simulink model "OcularMotorLabModel_2023_12_15_M22b"  (R2022b)
settings: Solver=FixedStepAuto  StartTime=tStart  StopTime=tFinal  FixedStep=0.001  RelTol=1e-3
undefined symbols (not defined in the file or in its folder): Asp, Asp1, Asp2, e0sp, gaussian, Gpc, GPos, Gsl, HeadToEye, IPD, psi, Psp1, RotFbk, SacThDeg, SatSp, sigbuilder_block, SomFbk, T1, T2, Tccanal, Tcn, Tcr, Tcsp, TCvs, tdm, tdsp1, tdsp2, tdsp3, tdv, Tsl, Tz, w
libraries: matrix_library x13, vrlib x9, simulink_extras x6, simulink x1
(part 2 of 2)

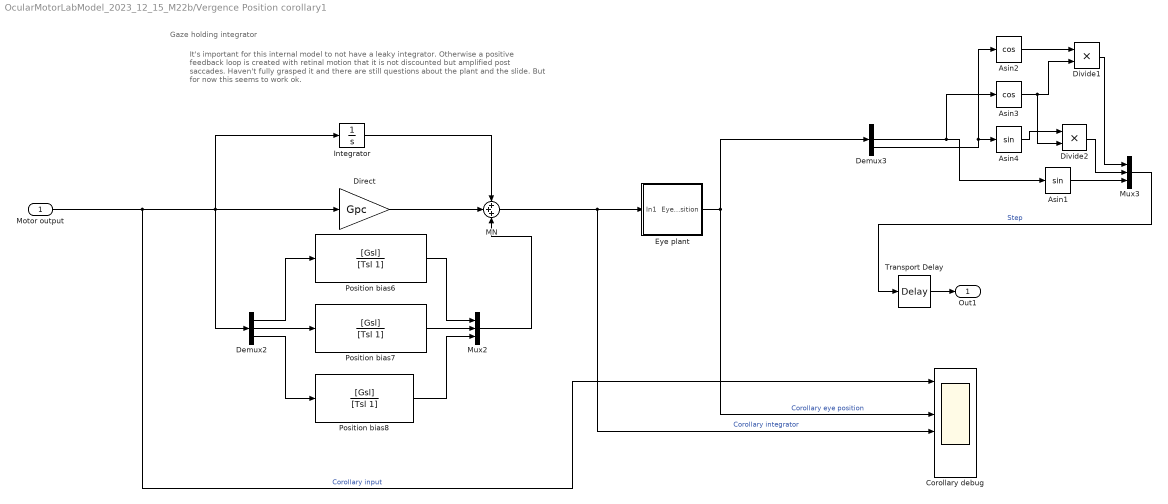
== system OcularMotorLabModel_2023_12_15_M22b/Vergence Position corollary1 ==
  note: Gaze holding integrator
  note: It's important for this internal model to not have a leaky integrator. Otherwise a positive feedback loop is created with retinal motion that it is not discounted but amplified post saccades.
      |
      | Haven't fully grasped it and there are still questions about the plant and the slide. But for now this seems to work ok.
  Motor output : Inport
  Asin1 : Trigonometry
  Asin2 : Trigonometry  Operator=cos
  Asin3 : Trigonometry  Operator=cos
  Asin4 : Trigonometry
  Corollary debug : Scope  NumInputPorts=6
  Demux2 : Demux  Outputs=3
  Demux3 : Demux  Outputs=3
  Direct : Gain  Gain=Gpc
  Divide1 : Product  Inputs=**
  Divide2 : Product  Inputs=**
  Eye plant : Subsystem
  Integrator : Integrator
  "MN " : Sum  Inputs=+++  InputSameDT=on  SaturateOnIntegerOverflow=on  OutDataTypeStr=Inherit: Same as first input
  Mux2 : Mux  Inputs=3
  Mux3 : Mux  Inputs=3
  Position bias6 : TransferFcn  Numerator=[Gsl]  Denominator=[Tsl 1]
  Position bias7 : TransferFcn  Numerator=[Gsl]  Denominator=[Tsl 1]
  Position bias8 : TransferFcn  Numerator=[Gsl]  Denominator=[Tsl 1]
  Transport Delay : TransportDelay  DelayTime=tdm
  Out1 : Outport
  wires:
  Motor output/1 -> Integrator/1, Direct/1, Demux2/1, Corollary debug/1  "Corollary input"
  Eye plant/1(Eye position) -> Demux3/1, Corollary debug/3  "Corollary eye position"
  "MN "/1 -> Eye plant/1(In1), Corollary debug/4  "Corollary integrator"
  Transport Delay/1 -> Out1/1
  Mux2/1 -> "MN "/3
  Integrator/1 -> "MN "/1
  Demux2/2 -> Position bias7/1
  Position bias8/1 -> Mux2/3
  Demux2/3 -> Position bias8/1
  Position bias6/1 -> Mux2/1
  Demux2/1 -> Position bias6/1
  Position bias7/1 -> Mux2/2
  Direct/1 -> "MN "/2
  Divide1/1 -> Mux3/1
  Asin1/1 -> Mux3/3
  Demux3/2 -> Asin3/1, Asin1/1
  Divide2/1 -> Mux3/2
  Asin3/1 -> Divide2/2, Divide1/2
  Asin2/1 -> Divide1/1
  Asin4/1 -> Divide2/1
  Demux3/3 -> Asin2/1, Asin4/1
  Mux3/1 -> Transport Delay/1  "Step"

== system OcularMotorLabModel_2023_12_15_M22b/Version ==
  Left : Inport
  Right : Inport  Port=2
  Constant : Constant  Value=2
  Divide : Product  Inputs=*/
  Sum : Sum  Inputs=|++
  Out1 : Outport
  wires:
  Divide/1 -> Out1/1
  Sum/1 -> Divide/1
  Left/1 -> Sum/1
  Constant/1 -> Divide/2
  Right/1 -> Sum/2

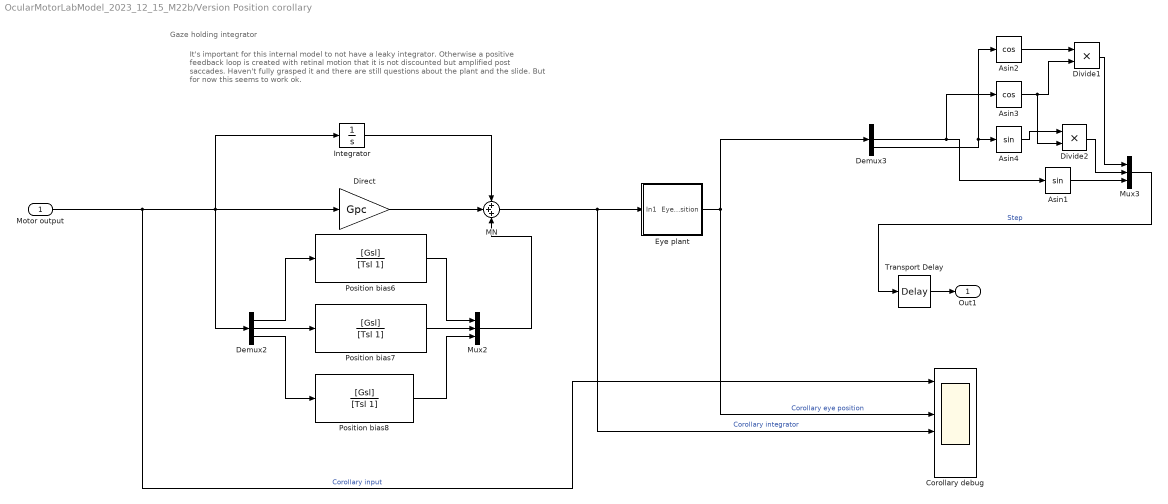
== system OcularMotorLabModel_2023_12_15_M22b/Version Position corollary ==
  note: Gaze holding integrator
  note: It's important for this internal model to not have a leaky integrator. Otherwise a positive feedback loop is created with retinal motion that it is not discounted but amplified post saccades.
      |
      | Haven't fully grasped it and there are still questions about the plant and the slide. But for now this seems to work ok.
  Motor output : Inport
  Asin1 : Trigonometry
  Asin2 : Trigonometry  Operator=cos
  Asin3 : Trigonometry  Operator=cos
  Asin4 : Trigonometry
  Corollary debug : Scope  NumInputPorts=6
  Demux2 : Demux  Outputs=3
  Demux3 : Demux  Outputs=3
  Direct : Gain  Gain=Gpc
  Divide1 : Product  Inputs=**
  Divide2 : Product  Inputs=**
  Eye plant : Subsystem
  Integrator : Integrator
  "MN " : Sum  Inputs=+++  InputSameDT=on  SaturateOnIntegerOverflow=on  OutDataTypeStr=Inherit: Same as first input
  Mux2 : Mux  Inputs=3
  Mux3 : Mux  Inputs=3
  Position bias6 : TransferFcn  Numerator=[Gsl]  Denominator=[Tsl 1]
  Position bias7 : TransferFcn  Numerator=[Gsl]  Denominator=[Tsl 1]
  Position bias8 : TransferFcn  Numerator=[Gsl]  Denominator=[Tsl 1]
  Transport Delay : TransportDelay  DelayTime=tdm
  Out1 : Outport
  wires:
  Motor output/1 -> Integrator/1, Direct/1, Demux2/1, Corollary debug/1  "Corollary input"
  Eye plant/1(Eye position) -> Demux3/1, Corollary debug/3  "Corollary eye position"
  "MN "/1 -> Eye plant/1(In1), Corollary debug/4  "Corollary integrator"
  Transport Delay/1 -> Out1/1
  Mux2/1 -> "MN "/3
  Integrator/1 -> "MN "/1
  Demux2/2 -> Position bias7/1
  Position bias8/1 -> Mux2/3
  Demux2/3 -> Position bias8/1
  Position bias6/1 -> Mux2/1
  Demux2/1 -> Position bias6/1
  Position bias7/1 -> Mux2/2
  Direct/1 -> "MN "/2
  Divide1/1 -> Mux3/1
  Asin1/1 -> Mux3/3
  Demux3/2 -> Asin3/1, Asin1/1
  Divide2/1 -> Mux3/2
  Asin3/1 -> Divide2/2, Divide1/2
  Asin2/1 -> Divide1/1
  Asin4/1 -> Divide2/1
  Demux3/3 -> Asin2/1, Asin4/1
  Mux3/1 -> Transport Delay/1  "Step"

== system OcularMotorLabModel_2023_12_15_M22b/Visual World Extrinsic Orientation (only for unidirectional reotations) ==
  Bus Creator : BusCreator  Tag=Bus Creator  Inputs=3
  FromWs : FromWorkspace  Tag=STV FromWs  VariableName=tuvar
      SigBuilderData=|
      | common.afterFinalStr = 'Extrapolate'
      | common.sampleTime = 0
      | dataSet(1).timeRange = [0 60]
      | dataSet(1).name = 'Roll 0.2 Hz'
      | dataSet(2).timeRange = [0 60]
      | dataSet(2).name = 'Roll 0.1 Hz'
      | dataSet(3).timeRange = [0 60]
      | dataSet(3).name = 'Roll 0.05 Hz'
      | dataSet(4).timeRange = [0 60]
      | dataSet(4).name = 'Roll 0.2 Hz IA'
      | dataSet(5).timeRange = [0 60]
      | dataSet(5).name = 'Roll 0.1 Hz IA'
      | dataSet(6).timeRange = [0 60]
      | dataSet(6).name = 'Roll 0.05 Hz IA'
      | dataSet(7).timeRange = [0 60]
      | dataSet(7).name = 'Roll 0.2 Hz RC'
      | dataSet(8).timeRange = [0 60]
      | dataSet(8).name = 'Roll 0.1 Hz RC'
      | dataSet(9).timeRange = [0 60]
      | dataSet(9).name = 'Roll 0.05 Hz RC'
      | dataSet(10).timeRange = [0 60]
      | dataSet(10).name = 'Zeros'
      | dataSet(11).timeRange = [0 60]
      | dataSet(11).name = 'SimpleSims'
      | sbobj.Groups(1).Name = 'Roll 0.2 Hz'
      | sbobj.Groups(1).Signals(1).Name = 'N-O (roll)'
      | sbobj.Groups(1).Signals(1).XData = [0 0.00500500500501 0.01001001001 0.015015015015 0.02002002002 0.025025025025 0.03003003003 0.035035035035 0.04004004004 0.045045045045 0.0500500500501 0.0550550550551 ... (11989 elements, 1x11989)]
      | sbobj.Groups(1).Signals(1).YData = [0 0.125788666321 0.251572356775 0.377346095689 0.503104907788 0.628843818382 0.754557853574 0.880242040448 1.00589140727 1.13150098368 1.25706580089 1.3825808919 ... (11989 elements, 1x11989)]
      | sbobj.Groups(1).Signals(2).Name = 'I-A (pitch)'
      | sbobj.Groups(1).Signals(2).XData = [0 60]
      | sbobj.Groups(1).Signals(2).YData = [0 0]
      | sbobj.Groups(1).Signals(3).Name = 'R-C (yaw)'
      | sbobj.Groups(1).Signals(3).XData = [0 60]
      | sbobj.Groups(1).Signals(3).YData = [0 0]
      | sbobj.Groups(1).TimeRange = [0 60]
      | sbobj.Groups(2).Name = 'Roll 0.1 Hz'
      | sbobj.Groups(2).Signals(1).Name = 'N-O (roll)'
      | sbobj.Groups(2).Signals(1).XData = [0 0.01001001001 0.02002002002 0.03003003003 0.04004004004 0.0500500500501 0.0600600600601 0.0700700700701 0.0800800800801 0.0900900900901 0.1001001001 0.11011011011 ... (5995 elements, 1x5995)]
      | sbobj.Groups(2).Signals(1).YData = [0 0.125788666321 0.251572356775 0.377346095689 0.503104907788 0.628843818382 0.754557853574 0.880242040448 1.00589140727 1.13150098368 1.25706580089 1.3825808919 ... (5995 elements, 1x5995)]
      | sbobj.Groups(2).Signals(2).Name = 'I-A (pitch)'
      | sbobj.Groups(2).Signals(2).XData = [0 60]
      | sbobj.Groups(2).Signals(2).YData = [0 0]
      | sbobj.Groups(2).Signals(3).Name = 'R-C (yaw)'
      | sbobj.Groups(2).Signals(3).XData = [0 60]
      | sbobj.Groups(2).Signals(3).YData = [0 0]
      | sbobj.Groups(2).TimeRange = [0 60]
      | sbobj.Groups(3).Name = 'Roll 0.05 Hz'
      | sbobj.Groups(3).Signals(1).Name = 'N-O (roll)'
      | sbobj.Groups(3).Signals(1).XData = [0 0.02002002002 0.04004004004 0.0600600600601 0.0800800800801 0.1001001001 0.12012012012 0.14014014014 0.16016016016 0.18018018018 0.2002002002 0.22022022022 ... (2998 elements, 1x2998)]
      | sbobj.Groups(3).Signals(1).YData = [0 0.125788666321 0.251572356775 0.377346095689 0.503104907788 0.628843818382 0.754557853574 0.880242040448 1.00589140727 1.13150098368 1.25706580089 1.3825808919 ... (2998 elements, 1x2998)]
      | sbobj.Groups(3).Signals(2).Name = 'I-A (pitch)'
      | sbobj.Groups(3).Signals(2).XData = [0 60]
      | sbobj.Groups(3).Signals(2).YData = [0 0]
      | sbobj.Groups(3).Signals(3).Name = 'R-C (yaw)'
      | sbobj.Groups(3).Signals(3).XData = [0 60]
      | sbobj.Groups(3).Signals(3).YData = [0 0]
      | sbobj.Groups(3).TimeRange = [0 60]
      | sbobj.Groups(4).Name = 'Roll 0.2 Hz IA'
      | sbobj.Groups(4).Signals(1).Name = 'N-O (roll)'
      | sbobj.Groups(4).Signals(1).XData = [0 60]
      | sbobj.Groups(4).Signals(1).YData = [0 0]
      | sbobj.Groups(4).Signals(2).Name = 'I-A (pitch)'
      | sbobj.Groups(4).Signals(2).XData = [0 0.00500500500501 0.01001001001 0.015015015015 0.02002002002 0.025025025025 0.03003003003 0.035035035035 0.04004004004 0.045045045045 0.0500500500501 0.0550550550551 ... (11989 elements, 1x11989)]
      | sbobj.Groups(4).Signals(2).YData = [0 0.125788666321 0.251572356775 0.377346095689 0.503104907788 0.628843818382 0.754557853574 0.880242040448 1.00589140727 1.13150098368 1.25706580089 1.3825808919 ... (11989 elements, 1x11989)]
      | sbobj.Groups(4).Signals(3).Name = 'R-C (yaw)'
      | sbobj.Groups(4).Signals(3).XData = [0 60]
      | sbobj.Groups(4).Signals(3).YData = [0 0]
      | sbobj.Groups(4).TimeRange = [0 60]
      | sbobj.Groups(5).Name = 'Roll 0.1 Hz IA'
      | sbobj.Groups(5).Signals(1).Name = 'N-O (roll)'
      | sbobj.Groups(5).Signals(1).XData = [0 60]
      | sbobj.Groups(5).Signals(1).YData = [0 0]
      | sbobj.Groups(5).Signals(2).Name = 'I-A (pitch)'
      | sbobj.Groups(5).Signals(2).XData = [0 0.01001001001 0.02002002002 0.03003003003 0.04004004004 0.0500500500501 0.0600600600601 0.0700700700701 0.0800800800801 0.0900900900901 0.1001001001 0.11011011011 ... (5995 elements, 1x5995)]
      | sbobj.Groups(5).Signals(2).YData = [0 0.125788666321 0.251572356775 0.377346095689 0.503104907788 0.628843818382 0.754557853574 0.880242040448 1.00589140727 1.13150098368 1.25706580089 1.3825808919 ... (5995 elements, 1x5995)]
      | sbobj.Groups(5).Signals(3).Name = 'R-C (yaw)'
      | sbobj.Groups(5).Signals(3).XData = [0 60]
      | sbobj.Groups(5).Signals(3).YData = [0 0]
      | sbobj.Groups(5).TimeRange = [0 60]
      | sbobj.Groups(6).Name = 'Roll 0.05 Hz IA'
      | sbobj.Groups(6).Signals(1).Name = 'N-O (roll)'
      | sbobj.Groups(6).Signals(1).XData = [0 60]
      | sbobj.Groups(6).Signals(1).YData = [0 0]
      | sbobj.Groups(6).Signals(2).Name = 'I-A (pitch)'
      | sbobj.Groups(6).Signals(2).XData = [0 0.02002002002 0.04004004004 0.0600600600601 0.0800800800801 0.1001001001 0.12012012012 0.14014014014 0.16016016016 0.18018018018 0.2002002002 0.22022022022 ... (2998 elements, 1x2998)]
      | sbobj.Groups(6).Signals(2).YData = [0 0.125788666321 0.251572356775 0.377346095689 0.503104907788 0.628843818382 0.754557853574 0.880242040448 1.00589140727 1.13150098368 1.25706580089 1.3825808919 ... (2998 elements, 1x2998)]
      | sbobj.Groups(6).Signals(3).Name = 'R-C (yaw)'
      | sbobj.Groups(6).Signals(3).XData = [0 60]
      | sbobj.Groups(6).Signals(3).YData = [0 0]
      | sbobj.Groups(6).TimeRange = [0 60]
      | sbobj.Groups(7).Name = 'Roll 0.2 Hz RC'
      | sbobj.Groups(7).Signals(1).Name = 'N-O (roll)'
      | sbobj.Groups(7).Signals(1).XData = [0 60]
      | sbobj.Groups(7).Signals(1).YData = [0 0]
      | sbobj.Groups(7).Signals(2).Name = 'I-A (pitch)'
      | sbobj.Groups(7).Signals(2).XData = [0 60]
      | sbobj.Groups(7).Signals(2).YData = [0 0]
      | sbobj.Groups(7).Signals(3).Name = 'R-C (yaw)'
      | sbobj.Groups(7).Signals(3).XData = [0 0.00500500500501 0.01001001001 0.015015015015 0.02002002002 0.025025025025 0.03003003003 0.035035035035 0.04004004004 0.045045045045 0.0500500500501 0.0550550550551 ... (11989 elements, 1x11989)]
      | sbobj.Groups(7).Signals(3).YData = [0 0.125788666321 0.251572356775 0.377346095689 0.503104907788 0.628843818382 0.754557853574 0.880242040448 1.00589140727 1.13150098368 1.25706580089 1.3825808919 ... (11989 elements, 1x11989)]
      | sbobj.Groups(7).TimeRange = [0 60]
      | sbobj.Groups(8).Name = 'Roll 0.1 Hz RC'
      | sbobj.Groups(8).Signals(1).Name = 'N-O (roll)'
      | sbobj.Groups(8).Signals(1).XData = [0 60]
      | sbobj.Groups(8).Signals(1).YData = [0 0]
      | sbobj.Groups(8).Signals(2).Name = 'I-A (pitch)'
      | sbobj.Groups(8).Signals(2).XData = [0 60]
      | sbobj.Groups(8).Signals(2).YData = [0 0]
      | sbobj.Groups(8).Signals(3).Name = 'R-C (yaw)'
      | sbobj.Groups(8).Signals(3).XData = [0 0.01001001001 0.02002002002 0.03003003003 0.04004004004 0.0500500500501 0.0600600600601 0.0700700700701 0.0800800800801 0.0900900900901 0.1001001001 0.11011011011 ... (5995 elements, 1x5995)]
      | sbobj.Groups(8).Signals(3).YData = [0 0.125788666321 0.251572356775 0.377346095689 0.503104907788 0.628843818382 0.754557853574 0.880242040448 1.00589140727 1.13150098368 1.25706580089 1.3825808919 ... (5995 elements, 1x5995)]
      | sbobj.Groups(8).TimeRange = [0 60]
      | sbobj.Groups(9).Name = 'Roll 0.05 Hz RC'
      | sbobj.Groups(9).Signals(1).Name = 'N-O (roll)'
      | sbobj.Groups(9).Signals(1).XData = [0 60]
      | sbobj.Groups(9).Signals(1).YData = [0 0]
      | sbobj.Groups(9).Signals(2).Name = 'I-A (pitch)'
      | sbobj.Groups(9).Signals(2).XData = [0 60]
      | sbobj.Groups(9).Signals(2).YData = [0 0]
      | sbobj.Groups(9).Signals(3).Name = 'R-C (yaw)'
      | sbobj.Groups(9).Signals(3).XData = [0 0.02002002002 0.04004004004 0.0600600600601 0.0800800800801 0.1001001001 0.12012012012 0.14014014014 0.16016016016 0.18018018018 0.2002002002 0.22022022022 ... (2998 elements, 1x2998)]
      | sbobj.Groups(9).Signals(3).YData = [0 0.125788666321 0.251572356775 0.377346095689 0.503104907788 0.628843818382 0.754557853574 0.880242040448 1.00589140727 1.13150098368 1.25706580089 1.3825808919 ... (2998 elements, 1x2998)]
      | sbobj.Groups(9).TimeRange = [0 60]
      | sbobj.Groups(10).Name = 'Zeros'
      | sbobj.Groups(10).Signals(1).Name = 'N-O (roll)'
      | sbobj.Groups(10).Signals(1).XData = [0 60]
      | sbobj.Groups(10).Signals(1).YData = [0 0]
      | sbobj.Groups(10).Signals(2).Name = 'I-A (pitch)'
      | sbobj.Groups(10).Signals(2).XData = [0 60]
      | sbobj.Groups(10).Signals(2).YData = [0 0]
      | sbobj.Groups(10).Signals(3).Name = 'R-C (yaw)'
      | sbobj.Groups(10).Signals(3).XData = [0 60]
      | sbobj.Groups(10).Signals(3).YData = [0 0]
      | sbobj.Groups(10).TimeRange = [0 60]
      | sbobj.Groups(11).Name = 'SimpleSims'
      | sbobj.Groups(11).Signals(1).Name = 'N-O (roll)'
      | sbobj.Groups(11).Signals(1).XData = [0 0.01 0.02 0.03 0.04 0.05 0.06 0.07 0.08 0.09 0.1 0.11 ... (6001 elements, 1x6001)]
      | sbobj.Groups(11).Signals(1).YData = [0 0.0628317497176 0.125662879311 0.188492768663 0.251320797667 0.314146346236 0.376968794308 0.43978752185 0.502601908867 0.565411335405 0.628215181563 0.691012827489 ... (6001 elements, 1x6001)]
      | sbobj.Groups(11).Signals(2).Name = 'I-A (pitch)'
      | sbobj.Groups(11).Signals(2).XData = [0 5 35 60]
      | sbobj.Groups(11).Signals(2).YData = [0 0 0 0]
      | sbobj.Groups(11).Signals(3).Name = 'R-C (yaw)'
      | sbobj.Groups(11).Signals(3).XData = [0 5 35 60]
      | sbobj.Groups(11).Signals(3).YData = [0 0 0 0]
      | sbobj.Groups(11).TimeRange = [0 60]
  Subsystem : Subsystem
  Bus : Outport
  wires:
  FromWs/1 -> Subsystem/1(In1)
  Subsystem/1(N-O (roll)) -> Bus Creator/1  "N-O (roll)"
  Subsystem/2(I-A (pitch)) -> Bus Creator/2  "I-A (pitch)"
  Subsystem/3(R-C (yaw)) -> Bus Creator/3  "R-C (yaw)"
  Bus Creator/1 -> Bus/1

== system OcularMotorLabModel_2023_12_15_M22b/Visual World Extrinsic velocity ==
  Bus Creator : BusCreator  Tag=Bus Creator  Inputs=3
  FromWs : FromWorkspace  Tag=STV FromWs  VariableName=tuvar
      SigBuilderData=|
      | common.afterFinalStr = 'Extrapolate'
      | common.sampleTime = 0
      | dataSet(1).timeRange = [0 60]
      | dataSet(1).name = 'Roll 0.2 Hz'
      | dataSet(2).timeRange = [0 60]
      | dataSet(2).name = 'Roll 0.1 Hz'
      | dataSet(3).timeRange = [0 60]
      | dataSet(3).name = 'Roll 0.05 Hz'
      | dataSet(4).timeRange = [0 60]
      | dataSet(4).name = 'Roll 0.2 Hz IA'
      | dataSet(5).timeRange = [0 60]
      | dataSet(5).name = 'Roll 0.1 Hz IA'
      | dataSet(6).timeRange = [0 60]
      | dataSet(6).name = 'Roll 0.05 Hz IA'
      | dataSet(7).timeRange = [0 60]
      | dataSet(7).name = 'Roll 0.2 Hz RC'
      | dataSet(8).timeRange = [0 60]
      | dataSet(8).name = 'Roll 0.1 Hz RC'
      | dataSet(9).timeRange = [0 60]
      | dataSet(9).name = 'Roll 0.05 Hz RC'
      | dataSet(10).timeRange = [0 60]
      | dataSet(10).name = 'Zeros'
      | dataSet(11).timeRange = [0 60]
      | dataSet(11).name = 'SimpleSims'
      | dataSet(12).timeRange = [0 60]
      | dataSet(12).name = 'YawOKN30degs'
      | sbobj.Groups(1).Name = 'Roll 0.2 Hz'
      | sbobj.Groups(1).Signals(1).Name = 'N-O (roll)'
      | sbobj.Groups(1).Signals(1).XData = [0 0.00500500500501 0.01001001001 0.015015015015 0.02002002002 0.025025025025 0.03003003003 0.035035035035 0.04004004004 0.045045045045 0.0500500500501 0.0550550550551 ... (11989 elements, 1x11989)]
      | sbobj.Groups(1).Signals(1).YData = [0 0.125788666321 0.251572356775 0.377346095689 0.503104907788 0.628843818382 0.754557853574 0.880242040448 1.00589140727 1.13150098368 1.25706580089 1.3825808919 ... (11989 elements, 1x11989)]
      | sbobj.Groups(1).Signals(2).Name = 'I-A (pitch)'
      | sbobj.Groups(1).Signals(2).XData = [0 60]
      | sbobj.Groups(1).Signals(2).YData = [0 0]
      | sbobj.Groups(1).Signals(3).Name = 'R-C (yaw)'
      | sbobj.Groups(1).Signals(3).XData = [0 60]
      | sbobj.Groups(1).Signals(3).YData = [0 0]
      | sbobj.Groups(1).TimeRange = [0 60]
      | sbobj.Groups(2).Name = 'Roll 0.1 Hz'
      | sbobj.Groups(2).Signals(1).Name = 'N-O (roll)'
      | sbobj.Groups(2).Signals(1).XData = [0 0.01001001001 0.02002002002 0.03003003003 0.04004004004 0.0500500500501 0.0600600600601 0.0700700700701 0.0800800800801 0.0900900900901 0.1001001001 0.11011011011 ... (5995 elements, 1x5995)]
      | sbobj.Groups(2).Signals(1).YData = [0 0.125788666321 0.251572356775 0.377346095689 0.503104907788 0.628843818382 0.754557853574 0.880242040448 1.00589140727 1.13150098368 1.25706580089 1.3825808919 ... (5995 elements, 1x5995)]
      | sbobj.Groups(2).Signals(2).Name = 'I-A (pitch)'
      | sbobj.Groups(2).Signals(2).XData = [0 60]
      | sbobj.Groups(2).Signals(2).YData = [0 0]
      | sbobj.Groups(2).Signals(3).Name = 'R-C (yaw)'
      | sbobj.Groups(2).Signals(3).XData = [0 60]
      | sbobj.Groups(2).Signals(3).YData = [0 0]
      | sbobj.Groups(2).TimeRange = [0 60]
      | sbobj.Groups(3).Name = 'Roll 0.05 Hz'
      | sbobj.Groups(3).Signals(1).Name = 'N-O (roll)'
      | sbobj.Groups(3).Signals(1).XData = [0 0.02002002002 0.04004004004 0.0600600600601 0.0800800800801 0.1001001001 0.12012012012 0.14014014014 0.16016016016 0.18018018018 0.2002002002 0.22022022022 ... (2998 elements, 1x2998)]
      | sbobj.Groups(3).Signals(1).YData = [0 0.125788666321 0.251572356775 0.377346095689 0.503104907788 0.628843818382 0.754557853574 0.880242040448 1.00589140727 1.13150098368 1.25706580089 1.3825808919 ... (2998 elements, 1x2998)]
      | sbobj.Groups(3).Signals(2).Name = 'I-A (pitch)'
      | sbobj.Groups(3).Signals(2).XData = [0 60]
      | sbobj.Groups(3).Signals(2).YData = [0 0]
      | sbobj.Groups(3).Signals(3).Name = 'R-C (yaw)'
      | sbobj.Groups(3).Signals(3).XData = [0 60]
      | sbobj.Groups(3).Signals(3).YData = [0 0]
      | sbobj.Groups(3).TimeRange = [0 60]
      | sbobj.Groups(4).Name = 'Roll 0.2 Hz IA'
      | sbobj.Groups(4).Signals(1).Name = 'N-O (roll)'
      | sbobj.Groups(4).Signals(1).XData = [0 60]
      | sbobj.Groups(4).Signals(1).YData = [0 0]
      | sbobj.Groups(4).Signals(2).Name = 'I-A (pitch)'
      | sbobj.Groups(4).Signals(2).XData = [0 0.00500500500501 0.01001001001 0.015015015015 0.02002002002 0.025025025025 0.03003003003 0.035035035035 0.04004004004 0.045045045045 0.0500500500501 0.0550550550551 ... (11989 elements, 1x11989)]
      | sbobj.Groups(4).Signals(2).YData = [0 0.125788666321 0.251572356775 0.377346095689 0.503104907788 0.628843818382 0.754557853574 0.880242040448 1.00589140727 1.13150098368 1.25706580089 1.3825808919 ... (11989 elements, 1x11989)]
      | sbobj.Groups(4).Signals(3).Name = 'R-C (yaw)'
      | sbobj.Groups(4).Signals(3).XData = [0 60]
      | sbobj.Groups(4).Signals(3).YData = [0 0]
      | sbobj.Groups(4).TimeRange = [0 60]
      | sbobj.Groups(5).Name = 'Roll 0.1 Hz IA'
      | sbobj.Groups(5).Signals(1).Name = 'N-O (roll)'
      | sbobj.Groups(5).Signals(1).XData = [0 60]
      | sbobj.Groups(5).Signals(1).YData = [0 0]
      | sbobj.Groups(5).Signals(2).Name = 'I-A (pitch)'
      | sbobj.Groups(5).Signals(2).XData = [0 0.01001001001 0.02002002002 0.03003003003 0.04004004004 0.0500500500501 0.0600600600601 0.0700700700701 0.0800800800801 0.0900900900901 0.1001001001 0.11011011011 ... (5995 elements, 1x5995)]
      | sbobj.Groups(5).Signals(2).YData = [0 0.125788666321 0.251572356775 0.377346095689 0.503104907788 0.628843818382 0.754557853574 0.880242040448 1.00589140727 1.13150098368 1.25706580089 1.3825808919 ... (5995 elements, 1x5995)]
      | sbobj.Groups(5).Signals(3).Name = 'R-C (yaw)'
      | sbobj.Groups(5).Signals(3).XData = [0 60]
      | sbobj.Groups(5).Signals(3).YData = [0 0]
      | sbobj.Groups(5).TimeRange = [0 60]
      | sbobj.Groups(6).Name = 'Roll 0.05 Hz IA'
      | sbobj.Groups(6).Signals(1).Name = 'N-O (roll)'
      | sbobj.Groups(6).Signals(1).XData = [0 60]
      | sbobj.Groups(6).Signals(1).YData = [0 0]
      | sbobj.Groups(6).Signals(2).Name = 'I-A (pitch)'
      | sbobj.Groups(6).Signals(2).XData = [0 0.02002002002 0.04004004004 0.0600600600601 0.0800800800801 0.1001001001 0.12012012012 0.14014014014 0.16016016016 0.18018018018 0.2002002002 0.22022022022 ... (2998 elements, 1x2998)]
      | sbobj.Groups(6).Signals(2).YData = [0 0.125788666321 0.251572356775 0.377346095689 0.503104907788 0.628843818382 0.754557853574 0.880242040448 1.00589140727 1.13150098368 1.25706580089 1.3825808919 ... (2998 elements, 1x2998)]
      | sbobj.Groups(6).Signals(3).Name = 'R-C (yaw)'
      | sbobj.Groups(6).Signals(3).XData = [0 60]
      | sbobj.Groups(6).Signals(3).YData = [0 0]
      | sbobj.Groups(6).TimeRange = [0 60]
      | sbobj.Groups(7).Name = 'Roll 0.2 Hz RC'
      | sbobj.Groups(7).Signals(1).Name = 'N-O (roll)'
      | sbobj.Groups(7).Signals(1).XData = [0 60]
      | sbobj.Groups(7).Signals(1).YData = [0 0]
      | sbobj.Groups(7).Signals(2).Name = 'I-A (pitch)'
      | sbobj.Groups(7).Signals(2).XData = [0 60]
      | sbobj.Groups(7).Signals(2).YData = [0 0]
      | sbobj.Groups(7).Signals(3).Name = 'R-C (yaw)'
      | sbobj.Groups(7).Signals(3).XData = [0 0.00500500500501 0.01001001001 0.015015015015 0.02002002002 0.025025025025 0.03003003003 0.035035035035 0.04004004004 0.045045045045 0.0500500500501 0.0550550550551 ... (11989 elements, 1x11989)]
      | sbobj.Groups(7).Signals(3).YData = [0 0.125788666321 0.251572356775 0.377346095689 0.503104907788 0.628843818382 0.754557853574 0.880242040448 1.00589140727 1.13150098368 1.25706580089 1.3825808919 ... (11989 elements, 1x11989)]
      | sbobj.Groups(7).TimeRange = [0 60]
      | sbobj.Groups(8).Name = 'Roll 0.1 Hz RC'
      | sbobj.Groups(8).Signals(1).Name = 'N-O (roll)'
      | sbobj.Groups(8).Signals(1).XData = [0 60]
      | sbobj.Groups(8).Signals(1).YData = [0 0]
      | sbobj.Groups(8).Signals(2).Name = 'I-A (pitch)'
      | sbobj.Groups(8).Signals(2).XData = [0 60]
      | sbobj.Groups(8).Signals(2).YData = [0 0]
      | sbobj.Groups(8).Signals(3).Name = 'R-C (yaw)'
      | sbobj.Groups(8).Signals(3).XData = [0 0.01001001001 0.02002002002 0.03003003003 0.04004004004 0.0500500500501 0.0600600600601 0.0700700700701 0.0800800800801 0.0900900900901 0.1001001001 0.11011011011 ... (5995 elements, 1x5995)]
      | sbobj.Groups(8).Signals(3).YData = [0 0.125788666321 0.251572356775 0.377346095689 0.503104907788 0.628843818382 0.754557853574 0.880242040448 1.00589140727 1.13150098368 1.25706580089 1.3825808919 ... (5995 elements, 1x5995)]
      | sbobj.Groups(8).TimeRange = [0 60]
      | sbobj.Groups(9).Name = 'Roll 0.05 Hz RC'
      | sbobj.Groups(9).Signals(1).Name = 'N-O (roll)'
      | sbobj.Groups(9).Signals(1).XData = [0 60]
      | sbobj.Groups(9).Signals(1).YData = [0 0]
      | sbobj.Groups(9).Signals(2).Name = 'I-A (pitch)'
      | sbobj.Groups(9).Signals(2).XData = [0 60]
      | sbobj.Groups(9).Signals(2).YData = [0 0]
      | sbobj.Groups(9).Signals(3).Name = 'R-C (yaw)'
      | sbobj.Groups(9).Signals(3).XData = [0 0.02002002002 0.04004004004 0.0600600600601 0.0800800800801 0.1001001001 0.12012012012 0.14014014014 0.16016016016 0.18018018018 0.2002002002 0.22022022022 ... (2998 elements, 1x2998)]
      | sbobj.Groups(9).Signals(3).YData = [0 0.125788666321 0.251572356775 0.377346095689 0.503104907788 0.628843818382 0.754557853574 0.880242040448 1.00589140727 1.13150098368 1.25706580089 1.3825808919 ... (2998 elements, 1x2998)]
      | sbobj.Groups(9).TimeRange = [0 60]
      | sbobj.Groups(10).Name = 'Zeros'
      | sbobj.Groups(10).Signals(1).Name = 'N-O (roll)'
      | sbobj.Groups(10).Signals(1).XData = [0 60]
      | sbobj.Groups(10).Signals(1).YData = [0 0]
      | sbobj.Groups(10).Signals(2).Name = 'I-A (pitch)'
      | sbobj.Groups(10).Signals(2).XData = [0 60]
      | sbobj.Groups(10).Signals(2).YData = [0 0]
      | sbobj.Groups(10).Signals(3).Name = 'R-C (yaw)'
      | sbobj.Groups(10).Signals(3).XData = [0 60]
      | sbobj.Groups(10).Signals(3).YData = [0 0]
      | sbobj.Groups(10).TimeRange = [0 60]
      | sbobj.Groups(11).Name = 'SimpleSims'
      | sbobj.Groups(11).Signals(1).Name = 'N-O (roll)'
      | sbobj.Groups(11).Signals(1).XData = [0 0.01 0.02 0.03 0.04 0.05 0.06 0.07 0.08 0.09 0.1 0.11 ... (6001 elements, 1x6001)]
      | sbobj.Groups(11).Signals(1).YData = [0 0.0628317497176 0.125662879311 0.188492768663 0.251320797667 0.314146346236 0.376968794308 0.43978752185 0.502601908867 0.565411335405 0.628215181563 0.691012827489 ... (6001 elements, 1x6001)]
      | sbobj.Groups(11).Signals(2).Name = 'I-A (pitch)'
      | sbobj.Groups(11).Signals(2).XData = [0 5 35 60]
      | sbobj.Groups(11).Signals(2).YData = [0 0 0 0]
      | sbobj.Groups(11).Signals(3).Name = 'R-C (yaw)'
      | sbobj.Groups(11).Signals(3).XData = [0 5 35 60]
      | sbobj.Groups(11).Signals(3).YData = [0 0 0 0]
      | sbobj.Groups(11).TimeRange = [0 60]
      | sbobj.Groups(12).Name = 'YawOKN30degs'
      | sbobj.Groups(12).Signals(1).Name = 'N-O (roll)'
      | sbobj.Groups(12).Signals(1).XData = [0 60]
      | sbobj.Groups(12).Signals(1).YData = [0 0]
      | sbobj.Groups(12).Signals(2).Name = 'I-A (pitch)'
      | sbobj.Groups(12).Signals(2).XData = [0 60]
      | sbobj.Groups(12).Signals(2).YData = [0 0]
      | sbobj.Groups(12).Signals(3).Name = 'R-C (yaw)'
      | sbobj.Groups(12).Signals(3).XData = [0 10 10 40.05 40.05 60]
      | sbobj.Groups(12).Signals(3).YData = [0 0 30 30 0 0]
      | sbobj.Groups(12).TimeRange = [0 60]
  Subsystem : Subsystem
  Bus : Outport
  wires:
  FromWs/1 -> Subsystem/1(In1)
  Subsystem/1(N-O (roll)) -> Bus Creator/1  "N-O (roll)"
  Subsystem/2(I-A (pitch)) -> Bus Creator/2  "I-A (pitch)"
  Subsystem/3(R-C (yaw)) -> Bus Creator/3  "R-C (yaw)"
  Bus Creator/1 -> Bus/1

== system OcularMotorLabModel_2023_12_15_M22b/Visual World Intrinsic velocity ==
  Bus Creator : BusCreator  Tag=Bus Creator  Inputs=3
  FromWs : FromWorkspace  Tag=STV FromWs  VariableName=tuvar
      SigBuilderData=|
      | common.afterFinalStr = 'Extrapolate'
      | common.sampleTime = 0
      | dataSet(1).timeRange = [0 60]
      | dataSet(1).name = 'Roll 0.2 Hz'
      | dataSet(2).timeRange = [0 60]
      | dataSet(2).name = 'Roll 0.1 Hz'
      | dataSet(3).timeRange = [0 60]
      | dataSet(3).name = 'Roll 0.05 Hz'
      | dataSet(4).timeRange = [0 60]
      | dataSet(4).name = 'Roll 0.2 Hz IA'
      | dataSet(5).timeRange = [0 60]
      | dataSet(5).name = 'Roll 0.1 Hz IA'
      | dataSet(6).timeRange = [0 60]
      | dataSet(6).name = 'Roll 0.05 Hz IA'
      | dataSet(7).timeRange = [0 60]
      | dataSet(7).name = 'Roll 0.2 Hz RC'
      | dataSet(8).timeRange = [0 60]
      | dataSet(8).name = 'Roll 0.1 Hz RC'
      | dataSet(9).timeRange = [0 60]
      | dataSet(9).name = 'Roll 0.05 Hz RC'
      | dataSet(10).timeRange = [0 60]
      | dataSet(10).name = 'Zeros'
      | dataSet(11).timeRange = [0 60]
      | dataSet(11).name = 'SimpleSims'
      | dataSet(12).timeRange = [0 60]
      | dataSet(12).name = 'YawOKN30degs'
      | sbobj.Groups(1).Name = 'Roll 0.2 Hz'
      | sbobj.Groups(1).Signals(1).Name = 'N-O (roll)'
      | sbobj.Groups(1).Signals(1).XData = [0 0.00500500500501 0.01001001001 0.015015015015 0.02002002002 0.025025025025 0.03003003003 0.035035035035 0.04004004004 0.045045045045 0.0500500500501 0.0550550550551 ... (11989 elements, 1x11989)]
      | sbobj.Groups(1).Signals(1).YData = [0 0.125788666321 0.251572356775 0.377346095689 0.503104907788 0.628843818382 0.754557853574 0.880242040448 1.00589140727 1.13150098368 1.25706580089 1.3825808919 ... (11989 elements, 1x11989)]
      | sbobj.Groups(1).Signals(2).Name = 'I-A (pitch)'
      | sbobj.Groups(1).Signals(2).XData = [0 60]
      | sbobj.Groups(1).Signals(2).YData = [0 0]
      | sbobj.Groups(1).Signals(3).Name = 'R-C (yaw)'
      | sbobj.Groups(1).Signals(3).XData = [0 60]
      | sbobj.Groups(1).Signals(3).YData = [0 0]
      | sbobj.Groups(1).TimeRange = [0 60]
      | sbobj.Groups(2).Name = 'Roll 0.1 Hz'
      | sbobj.Groups(2).Signals(1).Name = 'N-O (roll)'
      | sbobj.Groups(2).Signals(1).XData = [0 0.01001001001 0.02002002002 0.03003003003 0.04004004004 0.0500500500501 0.0600600600601 0.0700700700701 0.0800800800801 0.0900900900901 0.1001001001 0.11011011011 ... (5995 elements, 1x5995)]
      | sbobj.Groups(2).Signals(1).YData = [0 0.125788666321 0.251572356775 0.377346095689 0.503104907788 0.628843818382 0.754557853574 0.880242040448 1.00589140727 1.13150098368 1.25706580089 1.3825808919 ... (5995 elements, 1x5995)]
      | sbobj.Groups(2).Signals(2).Name = 'I-A (pitch)'
      | sbobj.Groups(2).Signals(2).XData = [0 60]
      | sbobj.Groups(2).Signals(2).YData = [0 0]
      | sbobj.Groups(2).Signals(3).Name = 'R-C (yaw)'
      | sbobj.Groups(2).Signals(3).XData = [0 60]
      | sbobj.Groups(2).Signals(3).YData = [0 0]
      | sbobj.Groups(2).TimeRange = [0 60]
      | sbobj.Groups(3).Name = 'Roll 0.05 Hz'
      | sbobj.Groups(3).Signals(1).Name = 'N-O (roll)'
      | sbobj.Groups(3).Signals(1).XData = [0 0.02002002002 0.04004004004 0.0600600600601 0.0800800800801 0.1001001001 0.12012012012 0.14014014014 0.16016016016 0.18018018018 0.2002002002 0.22022022022 ... (2998 elements, 1x2998)]
      | sbobj.Groups(3).Signals(1).YData = [0 0.125788666321 0.251572356775 0.377346095689 0.503104907788 0.628843818382 0.754557853574 0.880242040448 1.00589140727 1.13150098368 1.25706580089 1.3825808919 ... (2998 elements, 1x2998)]
      | sbobj.Groups(3).Signals(2).Name = 'I-A (pitch)'
      | sbobj.Groups(3).Signals(2).XData = [0 60]
      | sbobj.Groups(3).Signals(2).YData = [0 0]
      | sbobj.Groups(3).Signals(3).Name = 'R-C (yaw)'
      | sbobj.Groups(3).Signals(3).XData = [0 60]
      | sbobj.Groups(3).Signals(3).YData = [0 0]
      | sbobj.Groups(3).TimeRange = [0 60]
      | sbobj.Groups(4).Name = 'Roll 0.2 Hz IA'
      | sbobj.Groups(4).Signals(1).Name = 'N-O (roll)'
      | sbobj.Groups(4).Signals(1).XData = [0 60]
      | sbobj.Groups(4).Signals(1).YData = [0 0]
      | sbobj.Groups(4).Signals(2).Name = 'I-A (pitch)'
      | sbobj.Groups(4).Signals(2).XData = [0 0.00500500500501 0.01001001001 0.015015015015 0.02002002002 0.025025025025 0.03003003003 0.035035035035 0.04004004004 0.045045045045 0.0500500500501 0.0550550550551 ... (11989 elements, 1x11989)]
      | sbobj.Groups(4).Signals(2).YData = [0 0.125788666321 0.251572356775 0.377346095689 0.503104907788 0.628843818382 0.754557853574 0.880242040448 1.00589140727 1.13150098368 1.25706580089 1.3825808919 ... (11989 elements, 1x11989)]
      | sbobj.Groups(4).Signals(3).Name = 'R-C (yaw)'
      | sbobj.Groups(4).Signals(3).XData = [0 60]
      | sbobj.Groups(4).Signals(3).YData = [0 0]
      | sbobj.Groups(4).TimeRange = [0 60]
      | sbobj.Groups(5).Name = 'Roll 0.1 Hz IA'
      | sbobj.Groups(5).Signals(1).Name = 'N-O (roll)'
      | sbobj.Groups(5).Signals(1).XData = [0 60]
      | sbobj.Groups(5).Signals(1).YData = [0 0]
      | sbobj.Groups(5).Signals(2).Name = 'I-A (pitch)'
      | sbobj.Groups(5).Signals(2).XData = [0 0.01001001001 0.02002002002 0.03003003003 0.04004004004 0.0500500500501 0.0600600600601 0.0700700700701 0.0800800800801 0.0900900900901 0.1001001001 0.11011011011 ... (5995 elements, 1x5995)]
      | sbobj.Groups(5).Signals(2).YData = [0 0.125788666321 0.251572356775 0.377346095689 0.503104907788 0.628843818382 0.754557853574 0.880242040448 1.00589140727 1.13150098368 1.25706580089 1.3825808919 ... (5995 elements, 1x5995)]
      | sbobj.Groups(5).Signals(3).Name = 'R-C (yaw)'
      | sbobj.Groups(5).Signals(3).XData = [0 60]
      | sbobj.Groups(5).Signals(3).YData = [0 0]
      | sbobj.Groups(5).TimeRange = [0 60]
      | sbobj.Groups(6).Name = 'Roll 0.05 Hz IA'
      | sbobj.Groups(6).Signals(1).Name = 'N-O (roll)'
      | sbobj.Groups(6).Signals(1).XData = [0 60]
      | sbobj.Groups(6).Signals(1).YData = [0 0]
      | sbobj.Groups(6).Signals(2).Name = 'I-A (pitch)'
      | sbobj.Groups(6).Signals(2).XData = [0 0.02002002002 0.04004004004 0.0600600600601 0.0800800800801 0.1001001001 0.12012012012 0.14014014014 0.16016016016 0.18018018018 0.2002002002 0.22022022022 ... (2998 elements, 1x2998)]
      | sbobj.Groups(6).Signals(2).YData = [0 0.125788666321 0.251572356775 0.377346095689 0.503104907788 0.628843818382 0.754557853574 0.880242040448 1.00589140727 1.13150098368 1.25706580089 1.3825808919 ... (2998 elements, 1x2998)]
      | sbobj.Groups(6).Signals(3).Name = 'R-C (yaw)'
      | sbobj.Groups(6).Signals(3).XData = [0 60]
      | sbobj.Groups(6).Signals(3).YData = [0 0]
      | sbobj.Groups(6).TimeRange = [0 60]
      | sbobj.Groups(7).Name = 'Roll 0.2 Hz RC'
      | sbobj.Groups(7).Signals(1).Name = 'N-O (roll)'
      | sbobj.Groups(7).Signals(1).XData = [0 60]
      | sbobj.Groups(7).Signals(1).YData = [0 0]
      | sbobj.Groups(7).Signals(2).Name = 'I-A (pitch)'
      | sbobj.Groups(7).Signals(2).XData = [0 60]
      | sbobj.Groups(7).Signals(2).YData = [0 0]
      | sbobj.Groups(7).Signals(3).Name = 'R-C (yaw)'
      | sbobj.Groups(7).Signals(3).XData = [0 0.00500500500501 0.01001001001 0.015015015015 0.02002002002 0.025025025025 0.03003003003 0.035035035035 0.04004004004 0.045045045045 0.0500500500501 0.0550550550551 ... (11989 elements, 1x11989)]
      | sbobj.Groups(7).Signals(3).YData = [0 0.125788666321 0.251572356775 0.377346095689 0.503104907788 0.628843818382 0.754557853574 0.880242040448 1.00589140727 1.13150098368 1.25706580089 1.3825808919 ... (11989 elements, 1x11989)]
      | sbobj.Groups(7).TimeRange = [0 60]
      | sbobj.Groups(8).Name = 'Roll 0.1 Hz RC'
      | sbobj.Groups(8).Signals(1).Name = 'N-O (roll)'
      | sbobj.Groups(8).Signals(1).XData = [0 60]
      | sbobj.Groups(8).Signals(1).YData = [0 0]
      | sbobj.Groups(8).Signals(2).Name = 'I-A (pitch)'
      | sbobj.Groups(8).Signals(2).XData = [0 60]
      | sbobj.Groups(8).Signals(2).YData = [0 0]
      | sbobj.Groups(8).Signals(3).Name = 'R-C (yaw)'
      | sbobj.Groups(8).Signals(3).XData = [0 0.01001001001 0.02002002002 0.03003003003 0.04004004004 0.0500500500501 0.0600600600601 0.0700700700701 0.0800800800801 0.0900900900901 0.1001001001 0.11011011011 ... (5995 elements, 1x5995)]
      | sbobj.Groups(8).Signals(3).YData = [0 0.125788666321 0.251572356775 0.377346095689 0.503104907788 0.628843818382 0.754557853574 0.880242040448 1.00589140727 1.13150098368 1.25706580089 1.3825808919 ... (5995 elements, 1x5995)]
      | sbobj.Groups(8).TimeRange = [0 60]
      | sbobj.Groups(9).Name = 'Roll 0.05 Hz RC'
      | sbobj.Groups(9).Signals(1).Name = 'N-O (roll)'
      | sbobj.Groups(9).Signals(1).XData = [0 60]
      | sbobj.Groups(9).Signals(1).YData = [0 0]
      | sbobj.Groups(9).Signals(2).Name = 'I-A (pitch)'
      | sbobj.Groups(9).Signals(2).XData = [0 60]
      | sbobj.Groups(9).Signals(2).YData = [0 0]
      | sbobj.Groups(9).Signals(3).Name = 'R-C (yaw)'
      | sbobj.Groups(9).Signals(3).XData = [0 0.02002002002 0.04004004004 0.0600600600601 0.0800800800801 0.1001001001 0.12012012012 0.14014014014 0.16016016016 0.18018018018 0.2002002002 0.22022022022 ... (2998 elements, 1x2998)]
      | sbobj.Groups(9).Signals(3).YData = [0 0.125788666321 0.251572356775 0.377346095689 0.503104907788 0.628843818382 0.754557853574 0.880242040448 1.00589140727 1.13150098368 1.25706580089 1.3825808919 ... (2998 elements, 1x2998)]
      | sbobj.Groups(9).TimeRange = [0 60]
      | sbobj.Groups(10).Name = 'Zeros'
      | sbobj.Groups(10).Signals(1).Name = 'N-O (roll)'
      | sbobj.Groups(10).Signals(1).XData = [0 60]
      | sbobj.Groups(10).Signals(1).YData = [0 0]
      | sbobj.Groups(10).Signals(2).Name = 'I-A (pitch)'
      | sbobj.Groups(10).Signals(2).XData = [0 60]
      | sbobj.Groups(10).Signals(2).YData = [0 0]
      | sbobj.Groups(10).Signals(3).Name = 'R-C (yaw)'
      | sbobj.Groups(10).Signals(3).XData = [0 60]
      | sbobj.Groups(10).Signals(3).YData = [0 0]
      | sbobj.Groups(10).TimeRange = [0 60]
      | sbobj.Groups(11).Name = 'SimpleSims'
      | sbobj.Groups(11).Signals(1).Name = 'N-O (roll)'
      | sbobj.Groups(11).Signals(1).XData = [0 0.01 0.02 0.03 0.04 0.05 0.06 0.07 0.08 0.09 0.1 0.11 ... (6001 elements, 1x6001)]
      | sbobj.Groups(11).Signals(1).YData = [0 0.0628317497176 0.125662879311 0.188492768663 0.251320797667 0.314146346236 0.376968794308 0.43978752185 0.502601908867 0.565411335405 0.628215181563 0.691012827489 ... (6001 elements, 1x6001)]
      | sbobj.Groups(11).Signals(2).Name = 'I-A (pitch)'
      | sbobj.Groups(11).Signals(2).XData = [0 5 35 60]
      | sbobj.Groups(11).Signals(2).YData = [0 0 0 0]
      | sbobj.Groups(11).Signals(3).Name = 'R-C (yaw)'
      | sbobj.Groups(11).Signals(3).XData = [0 5 35 60]
      | sbobj.Groups(11).Signals(3).YData = [0 0 0 0]
      | sbobj.Groups(11).TimeRange = [0 60]
      | sbobj.Groups(12).Name = 'YawOKN30degs'
      | sbobj.Groups(12).Signals(1).Name = 'N-O (roll)'
      | sbobj.Groups(12).Signals(1).XData = [0 60]
      | sbobj.Groups(12).Signals(1).YData = [0 0]
      | sbobj.Groups(12).Signals(2).Name = 'I-A (pitch)'
      | sbobj.Groups(12).Signals(2).XData = [0 60]
      | sbobj.Groups(12).Signals(2).YData = [0 0]
      | sbobj.Groups(12).Signals(3).Name = 'R-C (yaw)'
      | sbobj.Groups(12).Signals(3).XData = [0 10 10 40.05 40.05 60]
      | sbobj.Groups(12).Signals(3).YData = [0 0 30 30 0 0]
      | sbobj.Groups(12).TimeRange = [0 60]
  Subsystem : Subsystem
  Bus : Outport
  wires:
  FromWs/1 -> Subsystem/1(In1)
  Subsystem/1(N-O (roll)) -> Bus Creator/1  "N-O (roll)"
  Subsystem/2(I-A (pitch)) -> Bus Creator/2  "I-A (pitch)"
  Subsystem/3(R-C (yaw)) -> Bus Creator/3  "R-C (yaw)"
  Bus Creator/1 -> Bus/1

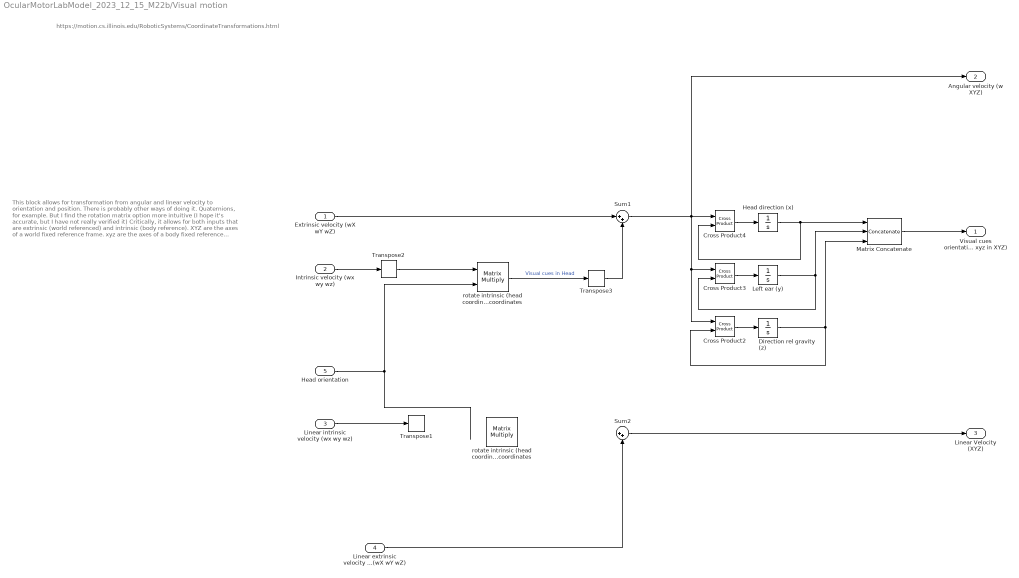
== system OcularMotorLabModel_2023_12_15_M22b/Visual motion ==
  note: https://motion.cs.illinois.edu/RoboticSystems/CoordinateTransformations.html
  note: This block allows for transformation from angular and linear velocity to orientation and position. There is probably other ways of doing it. Quaternions, for example. But I find the rotation matrix option more intuitive (I hope it's accurate, but I have not really verified it)
      |
      | Critically, it allows for both inputs that are extrinsic (world referenced) and intrinsic (body reference).
      |
      | XYZ are the axes of a world fixed reference frame.
      | xyz are the axes of a body fixed reference frame
      |
      | For the extrinsic angular velocities, they need to be integrated after a cross product with each of the xyz axis, that way they provide the rotation of such axis within the XYZ world fixed reference frame.
      |
      | For the intrinsic angular velocities, they simply multiply each of the intrisic axis and get added to the extrinsic velocities.
      |
      | A similar approach is followed for the linear velocities but without the cross products are linear velocities can be simply integrated by components.
  Extrinsic velocity (wX wY wZ) : Inport
  Intrinsic velocity (wx wy wz) : Inport  Port=2
  Linear intrinsic velocity (wx wy wz) : Inport  Port=3
  Linear extrinsic velocity (wX wY wZ) : Inport  Port=4
  Head orientation : Inport  Port=5
  Cross Product2 : vrlib/Utilities/Cross Product
  Cross Product3 : vrlib/Utilities/Cross Product
  Cross Product4 : vrlib/Utilities/Cross Product
  Direction rel gravity (z) : Integrator  InitialCondition=[0 0 1]'
  Head direction (x) : Integrator  InitialCondition=[1 0 0]'
  Left ear (y) : Integrator  InitialCondition=[0 1 0]'
  Matrix Concatenate : Concatenate  NumInputs=3  Mode=Multidimensional array  ConcatenateDimension=2
  Sum1 : Sum  Inputs=|++
  Sum2 : Sum  Inputs=|++
  Transpose1 : matrix_library/Transpose
  Transpose2 : matrix_library/Transpose
  Transpose3 : matrix_library/Transpose
  rotate intrinsic (head coordinates) linear motion vector to world coordinates : Product  Multiplication=Matrix(*)
  rotate intrinsic (head coordinates) rotation axis to world coordinates : Product  Multiplication=Matrix(*)
  Visual cues orientation in world (R xyz in XYZ) : Outport
  Angular velocity (w XYZ) : Outport  Port=2
  Linear Velocity (XYZ) : Outport  Port=3
  wires:
  Head direction (x)/1 -> Cross Product4/2, Matrix Concatenate/1
  Cross Product4/1 -> Head direction (x)/1
  Direction rel gravity (z)/1 -> Matrix Concatenate/3, Cross Product2/2
  Cross Product2/1 -> Direction rel gravity (z)/1
  Left ear (y)/1 -> Matrix Concatenate/2, Cross Product3/2
  Sum1/1 -> Angular velocity (w XYZ)/1, Cross Product2/1, Cross Product3/1, Cross Product4/1
  Cross Product3/1 -> Left ear (y)/1
  Matrix Concatenate/1 -> Visual cues orientation in world (R xyz in XYZ)/1
  Sum2/1 -> Linear Velocity (XYZ)/1
  Linear extrinsic velocity (wX wY wZ)/1 -> Sum2/2
  Extrinsic velocity (wX wY wZ)/1 -> Sum1/1
  Head orientation/1 -> rotate intrinsic (head coordinates) rotation axis to world coordinates/2
  Intrinsic velocity (wx wy wz)/1 -> Transpose2/1
  Transpose2/1 -> rotate intrinsic (head coordinates) rotation axis to world coordinates/1
  rotate intrinsic (head coordinates) rotation axis to world coordinates/1 -> Transpose3/1  "Visual cues in Head"
  Linear intrinsic velocity (wx wy wz)/1 -> Transpose1/1
  Transpose3/1 -> Sum1/2

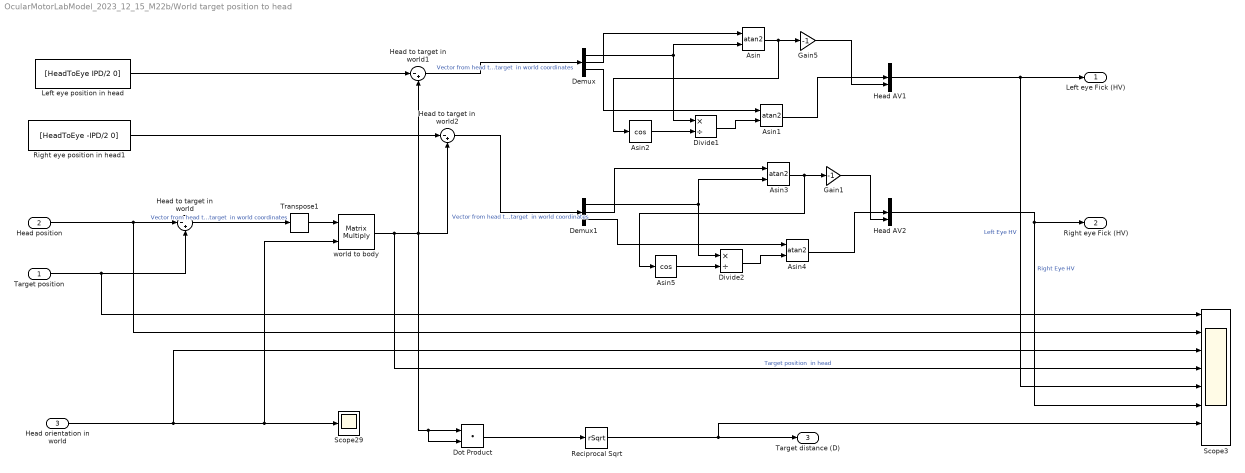
== system OcularMotorLabModel_2023_12_15_M22b/World target position to head ==
  Target position : Inport
  Head position : Inport  Port=2
  Head orientation in world : Inport  Port=3
  Asin{,1,3..4} (4 alike) : Trigonometry  Operator=atan2
  Asin2 : Trigonometry  Operator=cos
  Asin5 : Trigonometry  Operator=cos
  Demux : Demux  Outputs=3
  Demux1 : Demux  Outputs=3
  Divide1 : Product  Inputs=*/
  Divide2 : Product  Inputs=*/
  Dot Product : DotProduct  OutDataTypeStr=Inherit: Inherit via internal rule
  Gain1 : Gain  Gain=-1
  Gain5 : Gain  Gain=-1
  Head AV1 : Mux  Inputs=3
  Head AV2 : Mux  Inputs=3
  Head to target in world : Sum  Inputs=|-+
  Head to target in world1 : Sum  Inputs=|-+
  Head to target in world2 : Sum  Inputs=|-+
  Left eye position in head : Constant  Value=[HeadToEye IPD/2 0]
  Reciprocal Sqrt : Sqrt  Operator=rSqrt
  Right eye position in head1 : Constant  Value=[HeadToEye -IPD/2 0]
  Scope29 : Scope
  Scope3 : Scope  NumInputPorts=8
  Transpose1 : matrix_library/Transpose
  world to body : Product  Multiplication=Matrix(*)
  Left eye Fick (HV) : Outport
  Right eye Fick (HV) : Outport  Port=2
  Target distance (D) : Outport  Port=3
  wires:
  world to body/1 -> Scope3/4, Head to target in world1/2, Head to target in world2/2, Dot Product/2, Dot Product/1  "Target position  in head"
  Target position/1 -> Scope3/1, Head to target in world/2
  Head position/1 -> Scope3/2, Head to target in world/1
  Head to target in world/1 -> Transpose1/1  "Vector from head to target  in world coordinates"
  Head orientation in world/1 -> Scope3/3, world to body/2, Scope29/1
  Asin/1 -> Asin2/1, Gain5/1
  Transpose1/1 -> world to body/1
  Dot Product/1 -> Reciprocal Sqrt/1
  Reciprocal Sqrt/1 -> Scope3/7, Target distance (D)/1
  Head AV1/1 -> Scope3/5, Left eye Fick (HV)/1  "Left Eye HV"
  Left eye position in head/1 -> Head to target in world1/1
  Head to target in world1/1 -> Demux/1  "Vector from head to target  in world coordinates"
  Head AV2/1 -> Scope3/6, Right eye Fick (HV)/1  "Right Eye HV"
  Head to target in world2/1 -> Demux1/1  "Vector from head to target  in world coordinates"
  Right eye position in head1/1 -> Head to target in world2/1
  Demux/1 -> Asin/2, Divide1/1
  Demux/2 -> Asin/1
  Gain5/1 -> Head AV1/3
  Asin1/1 -> Head AV1/2
  Demux/3 -> Asin1/1
  Divide1/1 -> Asin1/2
  Asin2/1 -> Divide1/2
  Divide2/1 -> Asin4/2
  Demux1/2 -> Asin3/1
  Demux1/1 -> Asin3/2, Divide2/1
  Asin4/1 -> Head AV2/2
  Gain1/1 -> Head AV2/3
  Asin5/1 -> Divide2/2
  Asin3/1 -> Asin5/1, Gain1/1
  Demux1/3 -> Asin4/1

== system OcularMotorLabModel_2023_12_15_M22b/World to head ==
  note: GIa is calculated as the vector sum of G and linear acceleration in body reference
  Orientation : Inport
  Linear acceleration : Inport  Port=2
  1/G : Gain  Gain=1/9.8
  G (XYZ) : Constant  Value=[0 0 -1]  VectorParams1D=off
  Rotate gravity to body coordinates : Product  Multiplication=Matrix(*)
  Rotate gravity to body coordinates1 : Product  Multiplication=Matrix(*)
  Sum : Sum  Inputs=++|
  Transpose : matrix_library/Transpose
  Transpose1 : matrix_library/Transpose
  Transpose2 : matrix_library/Transpose
  GIA (in Gs) : Outport
  wires:
  Linear acceleration/1 -> Transpose/1
  Orientation/1 -> Rotate gravity to body coordinates/2, Rotate gravity to body coordinates1/2
  Rotate gravity to body coordinates/1 -> Transpose1/1
  G (XYZ)/1 -> Rotate gravity to body coordinates/1
  Sum/1 -> GIA (in Gs)/1  "GIA"
  1/G/1 -> Rotate gravity to body coordinates1/1
  Rotate gravity to body coordinates1/1 -> Transpose2/1
  Transpose/1 -> 1/G/1
  Transpose1/1 -> Sum/1
  Transpose2/1 -> Sum/2

== system OcularMotorLabModel_2023_12_15_M22b/World to head  ==
  Head orientation : Inport
  Head velocity : Inport  Port=2
  Transpose1 : matrix_library/Transpose
  world to body : Product  Multiplication=Matrix(*)
  Head velocity1 : Outport
  wires:
  Head orientation/1 -> world to body/2
  Head velocity/1 -> Transpose1/1
  Transpose1/1 -> world to body/1
  world to body/1 -> Head velocity1/1  "Head velocity"

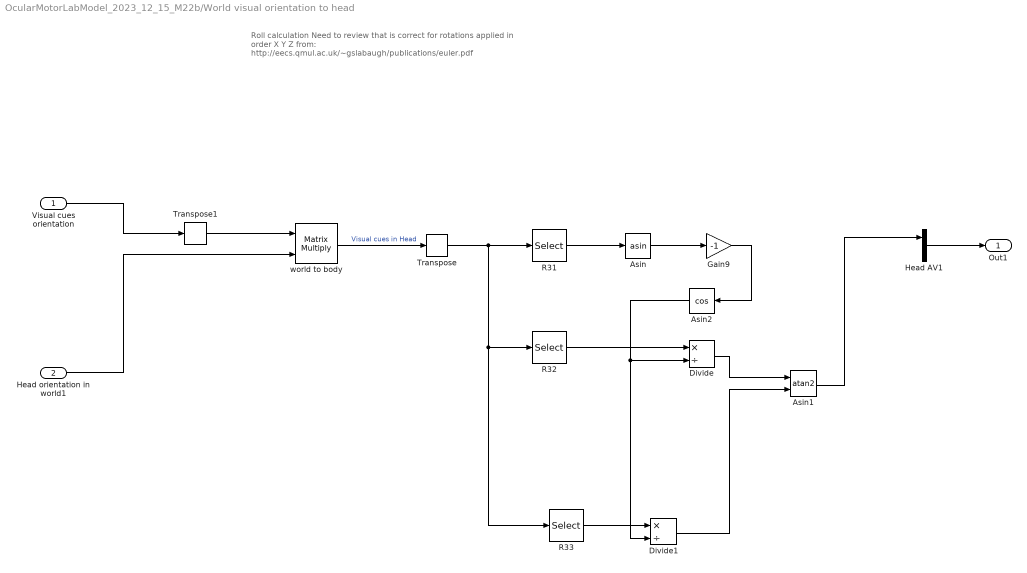
== system OcularMotorLabModel_2023_12_15_M22b/World visual orientation to head ==
  note: Roll calculation
      |
      | Need to review that is correct for rotations applied in order X Y Z
      |
      | from: http://eecs.qmul.ac.uk/~gslabaugh/publications/euler.pdf
  Visual cues orientation : Inport
  Head orientation in world1 : Inport  Port=2
  Asin : Trigonometry  Operator=asin
  Asin1 : Trigonometry  Operator=atan2
  Asin2 : Trigonometry  Operator=cos
  Divide : Product  Inputs=*/
  Divide1 : Product  Inputs=*/
  Gain9 : Gain  Gain=-1
  Head AV1 : Mux  Inputs=3
  R31 : Selector  NumberOfDimensions=2  InputPortWidth=3  IndexOptions=Index vector (dialog),Index vector (dialog)  Indices=3,1  OutputSizes=1,1
  R32 : Selector  NumberOfDimensions=2  InputPortWidth=3  IndexOptions=Index vector (dialog),Index vector (dialog)  Indices=3,2  OutputSizes=1,1
  R33 : Selector  NumberOfDimensions=2  InputPortWidth=3  IndexOptions=Index vector (dialog),Index vector (dialog)  Indices=3,3  OutputSizes=1,1
  Transpose : matrix_library/Transpose
  Transpose1 : matrix_library/Transpose
  world to body : Product  Multiplication=Matrix(*)
  Out1 : Outport
  wires:
  Transpose/1 -> R31/1, R32/1, R33/1
  world to body/1 -> Transpose/1  "Visual cues in Head"
  Visual cues orientation/1 -> Transpose1/1
  Head orientation in world1/1 -> world to body/2
  Gain9/1 -> Asin2/1
  Asin1/1 -> Head AV1/1
  Head AV1/1 -> Out1/1
  R31/1 -> Asin/1
  R32/1 -> Divide/1
  Asin/1 -> Gain9/1
  R33/1 -> Divide1/1
  Divide1/1 -> Asin1/2
  Divide/1 -> Asin1/1
  Transpose1/1 -> world to body/1
  Asin2/1 -> Divide1/2, Divide/2

== system OcularMotorLabModel_2023_12_15_M22b/World visual velocity  to head ==
  Visual velocity in world : Inport
  Head orientation in world : Inport  Port=2
  Transpose : matrix_library/Transpose
  Transpose1 : matrix_library/Transpose
  world to body : Product  Multiplication=Matrix(*)
  Out1 : Outport
  wires:
  Head orientation in world/1 -> world to body/2
  Visual velocity in world/1 -> Transpose1/1
  world to body/1 -> Transpose/1  "Visual velocity in Head"
  Transpose1/1 -> world to body/1
  Transpose/1 -> Out1/1

== system OcularMotorLabModel_2023_12_15_M22b/Head velocity (body)/Subsystem ==
  In1 : Inport
  Demux : Demux  Tag=STV Demux  Outputs=3
      settings: DisplayOption=none
  nasooccipital : Outport  Tag=STV Outport
  interaural : Outport  Tag=STV Outport  Port=2
  rostrocaudal : Outport  Tag=STV Outport  Port=3
  wires:
  Demux/1 -> nasooccipital/1
  Demux/2 -> interaural/1
  Demux/3 -> rostrocaudal/1
  In1/1 -> Demux/1

== system OcularMotorLabModel_2023_12_15_M22b/Head velocity (world)/Subsystem ==
  In1 : Inport
  Demux : Demux  Tag=STV Demux  Outputs=3
      settings: DisplayOption=none
  x : Outport  Tag=STV Outport
  y : Outport  Tag=STV Outport  Port=2
  z : Outport  Tag=STV Outport  Port=3
  wires:
  Demux/1 -> x/1
  Demux/2 -> y/1
  Demux/3 -> z/1
  In1/1 -> Demux/1

== system OcularMotorLabModel_2023_12_15_M22b/Linear body velocity/Subsystem ==
  Demux : Demux  Tag=STV Demux  Outputs=3
      settings: DisplayOption=none

== system OcularMotorLabModel_2023_12_15_M22b/Linear world velocity/Subsystem ==
  Demux : Demux  Tag=STV Demux  Outputs=3
      settings: DisplayOption=none

== system OcularMotorLabModel_2023_12_15_M22b/Only for simulations of spv/Left eye plant1 ==
  In1 : Inport
  Demux : Demux  Outputs=3
  Mux : Mux  Inputs=3
  Plant1 : TransferFcn  Numerator=[Tz 1]  Denominator=[T1*T2 (T1+T2) 1]
  Plant2 : TransferFcn  Numerator=[w^2]  Denominator=[1 + 2*psi*w w^2]
  Plant3 : TransferFcn  Numerator=[Tz 1]  Denominator=[T1*T2 (T1+T2) 1]
  Plant4 : TransferFcn  Numerator=[w^2]  Denominator=[1 + 2*psi*w w^2]
  Plant5 : TransferFcn  Numerator=[Tz 1]  Denominator=[T1*T2 (T1+T2) 1]
  Plant6 : TransferFcn  Numerator=[w^2]  Denominator=[1 + 2*psi*w w^2]
  Saturation : Saturate  UpperLimit=50*pi/180  LowerLimit=-50*pi/180
  Eye position : Outport
  wires:
  In1/1 -> Demux/1
  Mux/1 -> Saturation/1  "Eye position"
  Plant4/1 -> Mux/1
  Plant2/1 -> Mux/2
  Plant6/1 -> Mux/3
  Demux/1 -> Plant3/1
  Demux/2 -> Plant1/1
  Demux/3 -> Plant5/1
  Saturation/1 -> Eye position/1
  Plant3/1 -> Plant4/1
  Plant1/1 -> Plant2/1
  Plant5/1 -> Plant6/1

== system OcularMotorLabModel_2023_12_15_M22b/Pursuit velocity corollary/Eye plant ==
  In1 : Inport
  Demux : Demux  Outputs=3
  Mux : Mux  Inputs=3
  Plant1 : TransferFcn  Numerator=[Tz 1]  Denominator=[T1*T2 (T1+T2) 1]
  Plant2 : TransferFcn  Numerator=[w^2]  Denominator=[1 + 2*psi*w w^2]
  Plant3 : TransferFcn  Numerator=[Tz 1]  Denominator=[T1*T2 (T1+T2) 1]
  Plant4 : TransferFcn  Numerator=[w^2]  Denominator=[1 + 2*psi*w w^2]
  Plant5 : TransferFcn  Numerator=[Tz 1]  Denominator=[T1*T2 (T1+T2) 1]
  Plant6 : TransferFcn  Numerator=[w^2]  Denominator=[1 + 2*psi*w w^2]
  Eye position : Outport
  wires:
  In1/1 -> Demux/1
  Mux/1 -> Eye position/1  "Eye position"
  Plant4/1 -> Mux/1
  Plant2/1 -> Mux/2
  Plant6/1 -> Mux/3
  Demux/1 -> Plant3/1
  Demux/2 -> Plant1/1
  Demux/3 -> Plant5/1
  Plant3/1 -> Plant4/1
  Plant1/1 -> Plant2/1
  Plant5/1 -> Plant6/1

== system OcularMotorLabModel_2023_12_15_M22b/Saccade velocity corollary/Eye plant ==
  In1 : Inport
  Demux : Demux  Outputs=3
  Mux : Mux  Inputs=3
  Plant1 : TransferFcn  Numerator=[Tz 1]  Denominator=[T1*T2 (T1+T2) 1]
  Plant2 : TransferFcn  Numerator=[w^2]  Denominator=[1 + 2*psi*w w^2]
  Plant3 : TransferFcn  Numerator=[Tz 1]  Denominator=[T1*T2 (T1+T2) 1]
  Plant4 : TransferFcn  Numerator=[w^2]  Denominator=[1 + 2*psi*w w^2]
  Plant5 : TransferFcn  Numerator=[Tz 1]  Denominator=[T1*T2 (T1+T2) 1]
  Plant6 : TransferFcn  Numerator=[w^2]  Denominator=[1 + 2*psi*w w^2]
  Eye position : Outport
  wires:
  In1/1 -> Demux/1
  Mux/1 -> Eye position/1  "Eye position"
  Plant4/1 -> Mux/1
  Plant2/1 -> Mux/2
  Plant6/1 -> Mux/3
  Demux/1 -> Plant3/1
  Demux/2 -> Plant1/1
  Demux/3 -> Plant5/1
  Plant3/1 -> Plant4/1
  Plant1/1 -> Plant2/1
  Plant5/1 -> Plant6/1

== system OcularMotorLabModel_2023_12_15_M22b/Smooth pursuit/Left eye plant ==
  In1 : Inport
  Demux : Demux  Outputs=3
  Mux : Mux  Inputs=3
  Plant1 : TransferFcn  Numerator=[Tz 1]  Denominator=[T1*T2 (T1+T2) 1]
  Plant2 : TransferFcn  Numerator=[w^2]  Denominator=[1 + 2*psi*w w^2]
  Plant3 : TransferFcn  Numerator=[Tz 1]  Denominator=[T1*T2 (T1+T2) 1]
  Plant4 : TransferFcn  Numerator=[w^2]  Denominator=[1 + 2*psi*w w^2]
  Plant5 : TransferFcn  Numerator=[Tz 1]  Denominator=[T1*T2 (T1+T2) 1]
  Plant6 : TransferFcn  Numerator=[w^2]  Denominator=[1 + 2*psi*w w^2]
  Eye position : Outport
  wires:
  In1/1 -> Demux/1
  Mux/1 -> Eye position/1  "Eye position"
  Plant4/1 -> Mux/1
  Plant2/1 -> Mux/2
  Plant6/1 -> Mux/3
  Demux/1 -> Plant3/1
  Demux/2 -> Plant1/1
  Demux/3 -> Plant5/1
  Plant3/1 -> Plant4/1
  Plant1/1 -> Plant2/1
  Plant5/1 -> Plant6/1

== system OcularMotorLabModel_2023_12_15_M22b/Target position/Subsystem ==
  In1 : Inport
  Demux : Demux  Tag=STV Demux  Outputs=3
      settings: DisplayOption=none
  tX (m) : Outport  Tag=STV Outport  VectorParamsAs1DForOutWhenUnconnected=off
  tY (m) : Outport  Tag=STV Outport  Port=2  VectorParamsAs1DForOutWhenUnconnected=off
  tZ (m) : Outport  Tag=STV Outport  Port=3  VectorParamsAs1DForOutWhenUnconnected=off
  wires:
  Demux/1 -> tX (m)/1
  Demux/2 -> tY (m)/1
  Demux/3 -> tZ (m)/1
  In1/1 -> Demux/1

== system OcularMotorLabModel_2023_12_15_M22b/Vergence Position corollary1/Eye plant ==
  In1 : Inport
  Demux : Demux  Outputs=3
  Mux : Mux  Inputs=3
  Plant1 : TransferFcn  Numerator=[Tz 1]  Denominator=[T1*T2 (T1+T2) 1]
  Plant2 : TransferFcn  Numerator=[w^2]  Denominator=[1 + 2*psi*w w^2]
  Plant3 : TransferFcn  Numerator=[Tz 1]  Denominator=[T1*T2 (T1+T2) 1]
  Plant4 : TransferFcn  Numerator=[w^2]  Denominator=[1 + 2*psi*w w^2]
  Plant5 : TransferFcn  Numerator=[Tz 1]  Denominator=[T1*T2 (T1+T2) 1]
  Plant6 : TransferFcn  Numerator=[w^2]  Denominator=[1 + 2*psi*w w^2]
  Eye position : Outport
  wires:
  In1/1 -> Demux/1
  Mux/1 -> Eye position/1  "Eye position"
  Plant4/1 -> Mux/1
  Plant2/1 -> Mux/2
  Plant6/1 -> Mux/3
  Demux/1 -> Plant3/1
  Demux/2 -> Plant1/1
  Demux/3 -> Plant5/1
  Plant3/1 -> Plant4/1
  Plant1/1 -> Plant2/1
  Plant5/1 -> Plant6/1

== system OcularMotorLabModel_2023_12_15_M22b/Version Position corollary/Eye plant ==
  In1 : Inport
  Demux : Demux  Outputs=3
  Mux : Mux  Inputs=3
  Plant1 : TransferFcn  Numerator=[Tz 1]  Denominator=[T1*T2 (T1+T2) 1]
  Plant2 : TransferFcn  Numerator=[w^2]  Denominator=[1 + 2*psi*w w^2]
  Plant3 : TransferFcn  Numerator=[Tz 1]  Denominator=[T1*T2 (T1+T2) 1]
  Plant4 : TransferFcn  Numerator=[w^2]  Denominator=[1 + 2*psi*w w^2]
  Plant5 : TransferFcn  Numerator=[Tz 1]  Denominator=[T1*T2 (T1+T2) 1]
  Plant6 : TransferFcn  Numerator=[w^2]  Denominator=[1 + 2*psi*w w^2]
  Eye position : Outport
  wires:
  In1/1 -> Demux/1
  Mux/1 -> Eye position/1  "Eye position"
  Plant4/1 -> Mux/1
  Plant2/1 -> Mux/2
  Plant6/1 -> Mux/3
  Demux/1 -> Plant3/1
  Demux/2 -> Plant1/1
  Demux/3 -> Plant5/1
  Plant3/1 -> Plant4/1
  Plant1/1 -> Plant2/1
  Plant5/1 -> Plant6/1

== system OcularMotorLabModel_2023_12_15_M22b/Visual World Extrinsic Orientation (only for unidirectional reotations)/Subsystem ==
  In1 : Inport
  Demux : Demux  Tag=STV Demux  Outputs=3
      settings: DisplayOption=none
  N-O (roll) : Outport  Tag=STV Outport
  I-A (pitch) : Outport  Tag=STV Outport  Port=2
  R-C (yaw) : Outport  Tag=STV Outport  Port=3
  wires:
  Demux/1 -> N-O (roll)/1
  Demux/2 -> I-A (pitch)/1
  Demux/3 -> R-C (yaw)/1
  In1/1 -> Demux/1

== system OcularMotorLabModel_2023_12_15_M22b/Visual World Extrinsic velocity/Subsystem ==
  In1 : Inport
  Demux : Demux  Tag=STV Demux  Outputs=3
      settings: DisplayOption=none
  N-O (roll) : Outport  Tag=STV Outport
  I-A (pitch) : Outport  Tag=STV Outport  Port=2
  R-C (yaw) : Outport  Tag=STV Outport  Port=3
  wires:
  Demux/1 -> N-O (roll)/1
  Demux/2 -> I-A (pitch)/1
  Demux/3 -> R-C (yaw)/1
  In1/1 -> Demux/1

== system OcularMotorLabModel_2023_12_15_M22b/Visual World Intrinsic velocity/Subsystem ==
  In1 : Inport
  Demux : Demux  Tag=STV Demux  Outputs=3
      settings: DisplayOption=none
  N-O (roll) : Outport  Tag=STV Outport
  I-A (pitch) : Outport  Tag=STV Outport  Port=2
  R-C (yaw) : Outport  Tag=STV Outport  Port=3
  wires:
  Demux/1 -> N-O (roll)/1
  Demux/2 -> I-A (pitch)/1
  Demux/3 -> R-C (yaw)/1
  In1/1 -> Demux/1
